simulink model "CrCtl_ShOff"  (R2016b)
settings: configuration reference "CodeGenConfigSet" (kept outside this file)
values from neighbouring files (symbols this model uses):
  CrCtl_aAccShOff_C = Calibration.Parameter    [init_CrCtl_ShOff.m]
  CrCtl_aDeclShOff_C = Calibration.Parameter    [init_CrCtl_ShOff.m]
  CrCtl_facDvtRelShOff_C = Calibration.Parameter    [init_CrCtl_ShOff.m]
  CrCtl_GearMin_C = Calibration.Parameter    [init_CrCtl_ShOff.m]
  CrCtl_nMaxShOff_C = Calibration.Parameter    [init_CrCtl_ShOff.m]
  CrCtl_nMinShOff_C = Calibration.Parameter    [init_CrCtl_ShOff.m]
  CRCTL_PAUSEENABLE_SY = uint8(0)    [init_CrCtl_ShOff.m]
  CrCtl_rTraV2NDvtAbsShOff_C = Calibration.Parameter    [init_CrCtl_ShOff.m]
  CrCtl_rTraV2NDvtShOff_C = Calibration.Parameter    [init_CrCtl_ShOff.m]
  CrCtl_rTraV2NSuspSync_C = Calibration.Parameter    [init_CrCtl_ShOff.m]
  CrCtl_stShOffCut_C = Calibration.Parameter    [init_CrCtl_ShOff.m]
  CrCtl_stShOffIrvrs_C = Calibration.Parameter    [init_CrCtl_ShOff.m]
  CrCtl_stShOffRvrs_C = Calibration.Parameter    [init_CrCtl_ShOff.m]
  CrCtl_stShOffRvrsDelVel_C = Calibration.Parameter    [init_CrCtl_ShOff.m]
  CrCtl_stShOffSlpCnstRmp_C = Calibration.Parameter    [init_CrCtl_ShOff.m]
  CrCtl_stShOffTimeCnstRmp_C = Calibration.Parameter    [init_CrCtl_ShOff.m]
  CrCtl_swtSuspEna_C = Calibration.Parameter    [init_CrCtl_ShOff.m]
  CrCtl_tiAccShOff_C = Calibration.Parameter    [init_CrCtl_ShOff.m]
  CrCtl_tiDeclShOff_C = Calibration.Parameter    [init_CrCtl_ShOff.m]
  CrCtl_tiDvtShOff_C = Calibration.Parameter    [init_CrCtl_ShOff.m]
  CrCtl_tiOverrideShOff_C = Calibration.Parameter    [init_CrCtl_ShOff.m]
  CrCtl_tiSuspClthPresMax_C = Calibration.Parameter    [init_CrCtl_ShOff.m]
  CrCtl_tiSuspMax_C = Calibration.Parameter    [init_CrCtl_ShOff.m]
  CrCtl_tiSuspSync_C = Calibration.Parameter    [init_CrCtl_ShOff.m]
  CrCtl_trqSpdGovInc_C = Calibration.Parameter    [init_CrCtl_ShOff.m]
  CrCtl_trqSpdGovMax_C = Calibration.Parameter    [init_CrCtl_ShOff.m]
  CrCtl_trqSpdGovRed_C = Calibration.Parameter    [init_CrCtl_ShOff.m]
  CrCtl_vDvtNegShOff_C = Calibration.Parameter    [init_CrCtl_ShOff.m]
  CrCtl_vDvtPosShOff_C = Calibration.Parameter    [init_CrCtl_ShOff.m]
  CrCtl_vDvtShOff_C = Calibration.Parameter    [init_CrCtl_ShOff.m]
  CrCtl_vMaxShOff_C = Calibration.Parameter    [init_CrCtl_ShOff.m]
  CrCtl_vMinShOff_C = Calibration.Parameter    [init_CrCtl_ShOff.m]
  TRQ_ENGINTV_SY = uint8(1)    [init_CrCtl_ShOff.m]
  VEL_ZERO = fi(0,VehSpeed_km_h)    [init_CrCtl_ShOff.m]
undefined symbols (not defined in the file or in its folder): CrCtl_ShOff_DT, CrCtl_stLck_conv, CrCtl_stOpFunc_conv, CrCtl_stShOff_conv, CrCtl_stSub_conv, CrCUI_BttnState_conv, CruiseCtl_State_conv, EngState_conv, Switch_conv
libraries: simulink x80, CXLib x24
(part 2 of 2)

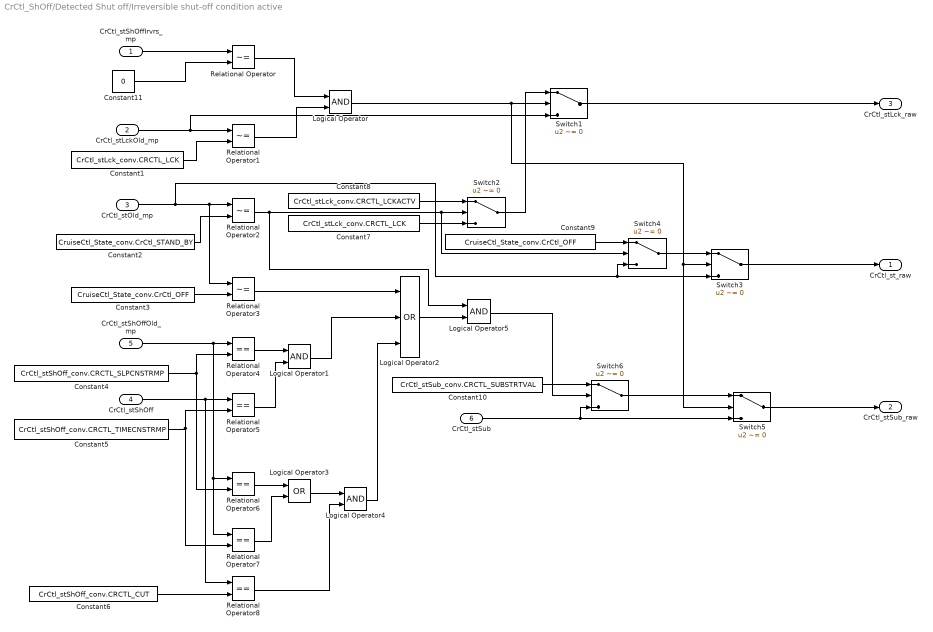
== system CrCtl_ShOff/Detected Shut off/Irreversible shut-off condition active ==
  CrCtl_stShOffIrvrs_mp : Inport
  CrCtl_stLckOld_mp : Inport  Port=2
  CrCtl_stOld_mp : Inport  Port=3
  CrCtl_stShOff : Inport  Port=4
  CrCtl_stShOffOld_mp : Inport  Port=5
  CrCtl_stSub : Inport  Port=6
  Constant1 : Constant  Value=CrCtl_stLck_conv.CRCTL_LCK
  Constant10 : Constant  Value=CrCtl_stSub_conv.CRCTL_SUBSTRTVAL
  Constant11 : Constant  Value=0  OutDataTypeStr=uint16
  Constant2 : Constant  Value=CruiseCtl_State_conv.CrCtl_STAND_BY
  Constant3 : Constant  Value=CruiseCtl_State_conv.CrCtl_OFF
  Constant4 : Constant  Value=CrCtl_stShOff_conv.CRCTL_SLPCNSTRMP
  Constant5 : Constant  Value=CrCtl_stShOff_conv.CRCTL_TIMECNSTRMP
  Constant6 : Constant  Value=CrCtl_stShOff_conv.CRCTL_CUT
  Constant7 : Constant  Value=CrCtl_stLck_conv.CRCTL_LCK
  Constant8 : Constant  Value=CrCtl_stLck_conv.CRCTL_LCKACTV
  Constant9 : Constant  Value=CruiseCtl_State_conv.CrCtl_OFF
  Logical Operator{,1,4..5} (4 alike) : Logic  AllPortsSameDT=off  OutDataTypeStr=boolean
  Logical Operator2 : Logic  Operator=OR  Inputs=3  AllPortsSameDT=off  OutDataTypeStr=boolean
  Logical Operator3 : Logic  Operator=OR  AllPortsSameDT=off  OutDataTypeStr=boolean
  Relational Operator{,1..3} (4 alike) : RelationalOperator  Operator=~=  OutDataTypeStr=boolean  RndMeth=Simplest
  Relational Operator{4..8} (5 alike) : RelationalOperator  Operator===  OutDataTypeStr=boolean  RndMeth=Simplest
  Switch{1..6} (6 alike) : Switch  Criteria=u2 ~= 0
  CrCtl_st_raw : Outport
  CrCtl_stSub_raw : Outport  Port=2
  CrCtl_stLck_raw : Outport  Port=3
  wires:
  CrCtl_stShOffIrvrs_mp/1 -> Relational Operator/1
  Constant11/1 -> Relational Operator/2
  Constant1/1 -> Relational Operator1/2
  Constant2/1 -> Relational Operator2/2
  Constant3/1 -> Relational Operator3/2
  CrCtl_stShOffOld_mp/1 -> Relational Operator7/1, Relational Operator6/1, Relational Operator4/1
  Constant4/1 -> Relational Operator6/2, Relational Operator4/2
  CrCtl_stShOff/1 -> Relational Operator8/1, Relational Operator5/1
  Constant5/1 -> Relational Operator7/2, Relational Operator5/2
  Constant6/1 -> Relational Operator8/2
  Relational Operator/1 -> Logical Operator/1
  Relational Operator1/1 -> Logical Operator/2
  Switch1/1 -> CrCtl_stLck_raw/1
  CrCtl_stLckOld_mp/1 -> Switch1/3, Relational Operator1/1
  Relational Operator2/1 -> Switch4/2, Switch2/2, Logical Operator5/1
  Switch2/1 -> Switch1/1
  Constant7/1 -> Switch2/3
  Constant8/1 -> Switch2/1
  Relational Operator4/1 -> Logical Operator1/1
  Relational Operator5/1 -> Logical Operator1/2
  Logical Operator1/1 -> Logical Operator2/2
  Relational Operator3/1 -> Logical Operator2/1
  Relational Operator6/1 -> Logical Operator3/1
  Relational Operator7/1 -> Logical Operator3/2
  Relational Operator8/1 -> Logical Operator4/2
  Logical Operator3/1 -> Logical Operator4/1
  Logical Operator4/1 -> Logical Operator2/3
  Logical Operator2/1 -> Logical Operator5/2
  Switch3/1 -> CrCtl_st_raw/1
  CrCtl_stOld_mp/1 -> Switch4/3, Switch3/3, Relational Operator3/1, Relational Operator2/1
  Switch4/1 -> Switch3/1
  Logical Operator/1 -> Switch5/2, Switch3/2, Switch1/2
  Switch5/1 -> CrCtl_stSub_raw/1
  CrCtl_stSub/1 -> Switch5/3, Switch6/3
  Switch6/1 -> Switch5/1
  Constant9/1 -> Switch4/1
  Logical Operator5/1 -> Switch6/2
  Constant10/1 -> Switch6/1

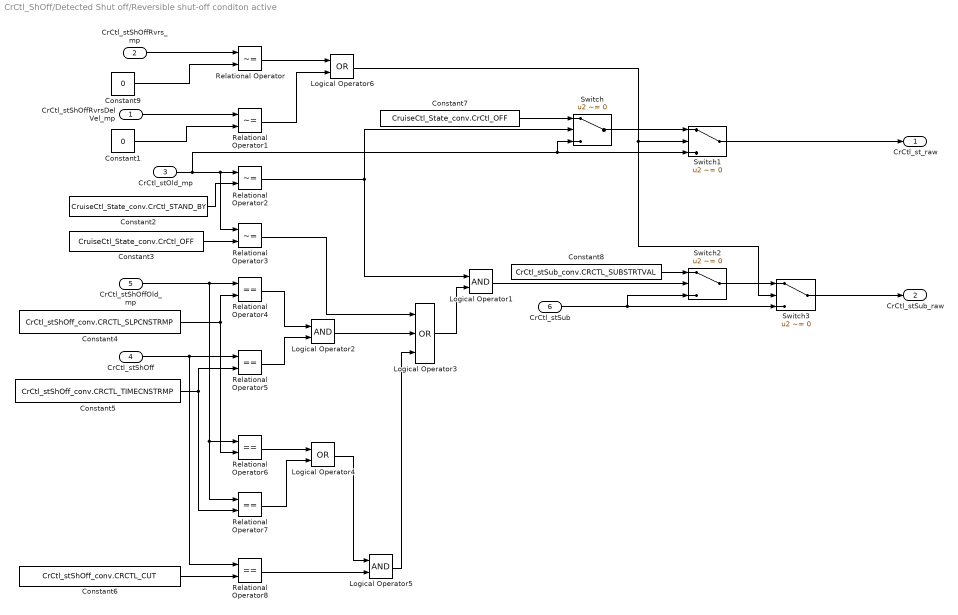
== system CrCtl_ShOff/Detected Shut off/Reversible shut-off conditon active ==
  CrCtl_stShOffRvrsDelVel_mp : Inport
  CrCtl_stShOffRvrs_mp : Inport  Port=2
  CrCtl_stOld_mp : Inport  Port=3
  CrCtl_stShOff : Inport  Port=4
  CrCtl_stShOffOld_mp : Inport  Port=5
  CrCtl_stSub : Inport  Port=6
  Constant1 : Constant  Value=0  OutDataTypeStr=uint16
  Constant2 : Constant  Value=CruiseCtl_State_conv.CrCtl_STAND_BY
  Constant3 : Constant  Value=CruiseCtl_State_conv.CrCtl_OFF
  Constant4 : Constant  Value=CrCtl_stShOff_conv.CRCTL_SLPCNSTRMP
  Constant5 : Constant  Value=CrCtl_stShOff_conv.CRCTL_TIMECNSTRMP
  Constant6 : Constant  Value=CrCtl_stShOff_conv.CRCTL_CUT
  Constant7 : Constant  Value=CruiseCtl_State_conv.CrCtl_OFF
  Constant8 : Constant  Value=CrCtl_stSub_conv.CRCTL_SUBSTRTVAL
  Constant9 : Constant  Value=0  OutDataTypeStr=uint16
  Logical Operator1 : Logic  AllPortsSameDT=off  OutDataTypeStr=boolean
  Logical Operator2 : Logic  AllPortsSameDT=off  OutDataTypeStr=boolean
  Logical Operator3 : Logic  Operator=OR  Inputs=3  AllPortsSameDT=off  OutDataTypeStr=boolean
  Logical Operator4 : Logic  Operator=OR  AllPortsSameDT=off  OutDataTypeStr=boolean
  Logical Operator5 : Logic  AllPortsSameDT=off  OutDataTypeStr=boolean
  Logical Operator6 : Logic  Operator=OR  AllPortsSameDT=off  OutDataTypeStr=boolean
  Relational Operator{,1..3} (4 alike) : RelationalOperator  Operator=~=  OutDataTypeStr=boolean  RndMeth=Simplest
  Relational Operator{4..8} (5 alike) : RelationalOperator  Operator===  OutDataTypeStr=boolean  RndMeth=Simplest
  Switch{,1..3} (4 alike) : Switch  Criteria=u2 ~= 0
  CrCtl_st_raw : Outport
  CrCtl_stSub_raw : Outport  Port=2
  wires:
  CrCtl_stShOffRvrs_mp/1 -> Relational Operator/1
  Constant9/1 -> Relational Operator/2
  CrCtl_stShOffRvrsDelVel_mp/1 -> Relational Operator1/1
  Constant1/1 -> Relational Operator1/2
  Constant2/1 -> Relational Operator2/2
  Constant3/1 -> Relational Operator3/2
  CrCtl_stShOffOld_mp/1 -> Relational Operator7/1, Relational Operator6/1, Relational Operator4/1
  Constant4/1 -> Relational Operator4/2, Relational Operator6/2
  CrCtl_stShOff/1 -> Relational Operator8/1, Relational Operator5/1
  Constant5/1 -> Relational Operator5/2, Relational Operator7/2
  Constant6/1 -> Relational Operator8/2
  Relational Operator/1 -> Logical Operator6/1
  Relational Operator1/1 -> Logical Operator6/2
  Relational Operator2/1 -> Logical Operator1/1, Switch/2
  Switch/1 -> Switch1/1
  Switch1/1 -> CrCtl_st_raw/1
  CrCtl_stOld_mp/1 -> Switch/3, Switch1/3, Relational Operator3/1, Relational Operator2/1
  Constant7/1 -> Switch/1
  Relational Operator4/1 -> Logical Operator2/1
  Relational Operator5/1 -> Logical Operator2/2
  Logical Operator2/1 -> Logical Operator3/2
  Relational Operator3/1 -> Logical Operator3/1
  Relational Operator6/1 -> Logical Operator4/1
  Relational Operator7/1 -> Logical Operator4/2
  Relational Operator8/1 -> Logical Operator5/2
  Logical Operator4/1 -> Logical Operator5/1
  Logical Operator5/1 -> Logical Operator3/3
  Logical Operator3/1 -> Logical Operator1/2
  Logical Operator1/1 -> Switch2/2
  Switch2/1 -> Switch3/1
  Switch3/1 -> CrCtl_stSub_raw/1
  CrCtl_stSub/1 -> Switch3/3, Switch2/3
  Constant8/1 -> Switch2/1
  Logical Operator6/1 -> Switch3/2, Switch1/2

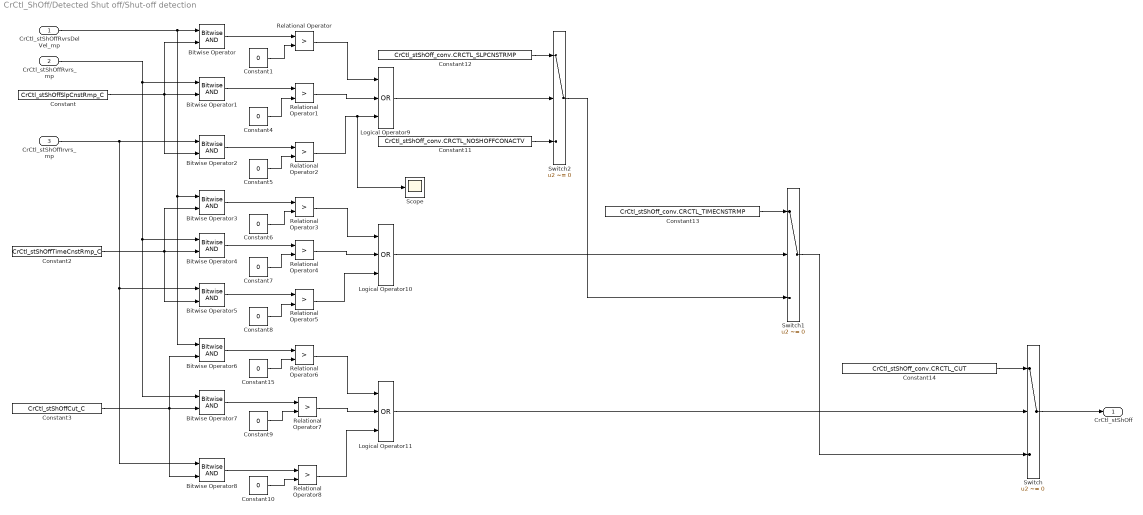
== system CrCtl_ShOff/Detected Shut off/Shut-off detection ==
  CrCtl_stShOffRvrsDelVel_mp : Inport
  CrCtl_stShOffRvrs_mp : Inport  Port=2
  CrCtl_stShOffIrvrs_mp : Inport  Port=3
  Bitwise Operator{,1..8} (9 alike) : simulink/Logic and Bit Operations/Bitwise Operator  logicop=AND  UseBitMask=off  NumInputPorts=2  BitMask=bin2dec('11011001')  BitMaskRealWorld=Stored Integer
  Constant : Constant  Value=CrCtl_stShOffSlpCnstRmp_C
  Constant{1,4..10,15} (9 alike) : Constant  Value=0  OutDataTypeStr=uint32
  Constant11 : Constant  Value=CrCtl_stShOff_conv.CRCTL_NOSHOFFCONACTV
  Constant12 : Constant  Value=CrCtl_stShOff_conv.CRCTL_SLPCNSTRMP
  Constant13 : Constant  Value=CrCtl_stShOff_conv.CRCTL_TIMECNSTRMP
  Constant14 : Constant  Value=CrCtl_stShOff_conv.CRCTL_CUT
  Constant2 : Constant  Value=CrCtl_stShOffTimeCnstRmp_C
  Constant3 : Constant  Value=CrCtl_stShOffCut_C
  Logical Operator10 : Logic  Operator=OR  Inputs=3  AllPortsSameDT=off  OutDataTypeStr=boolean
  Logical Operator11 : Logic  Operator=OR  Inputs=3  AllPortsSameDT=off  OutDataTypeStr=boolean
  Logical Operator9 : Logic  Operator=OR  Inputs=3  AllPortsSameDT=off  OutDataTypeStr=boolean
  Relational Operator{,1..8} (9 alike) : RelationalOperator  Operator=>  OutDataTypeStr=boolean  RndMeth=Simplest
  Scope : Scope
  Switch : Switch  Criteria=u2 ~= 0
  Switch1 : Switch  Criteria=u2 ~= 0
  Switch2 : Switch  Criteria=u2 ~= 0
  CrCtl_stShOff : Outport
  wires:
  Constant3/1 -> Bitwise Operator8/2, Bitwise Operator7/2, Bitwise Operator6/2
  CrCtl_stShOffRvrsDelVel_mp/1 -> Bitwise Operator6/1, Bitwise Operator3/1, Bitwise Operator/1
  CrCtl_stShOffRvrs_mp/1 -> Bitwise Operator7/1, Bitwise Operator4/1, Bitwise Operator1/1
  CrCtl_stShOffIrvrs_mp/1 -> Bitwise Operator8/1, Bitwise Operator5/1, Bitwise Operator2/1
  Constant/1 -> Bitwise Operator2/2, Bitwise Operator1/2, Bitwise Operator/2
  Constant2/1 -> Bitwise Operator5/2, Bitwise Operator4/2, Bitwise Operator3/2
  Constant1/1 -> Relational Operator/2
  Bitwise Operator/1 -> Relational Operator/1
  Bitwise Operator1/1 -> Relational Operator1/1
  Constant4/1 -> Relational Operator1/2
  Bitwise Operator2/1 -> Relational Operator2/1
  Constant5/1 -> Relational Operator2/2
  Bitwise Operator3/1 -> Relational Operator3/1
  Constant6/1 -> Relational Operator3/2
  Bitwise Operator4/1 -> Relational Operator4/1
  Constant7/1 -> Relational Operator4/2
  Bitwise Operator5/1 -> Relational Operator5/1
  Constant8/1 -> Relational Operator5/2
  Bitwise Operator6/1 -> Relational Operator6/1
  Constant15/1 -> Relational Operator6/2
  Bitwise Operator7/1 -> Relational Operator7/1
  Constant9/1 -> Relational Operator7/2
  Bitwise Operator8/1 -> Relational Operator8/1
  Constant10/1 -> Relational Operator8/2
  Relational Operator1/1 -> Logical Operator9/2
  Relational Operator/1 -> Logical Operator9/1
  Relational Operator2/1 -> Scope/1, Logical Operator9/3
  Relational Operator4/1 -> Logical Operator10/2
  Relational Operator3/1 -> Logical Operator10/1
  Relational Operator5/1 -> Logical Operator10/3
  Relational Operator7/1 -> Logical Operator11/2
  Relational Operator6/1 -> Logical Operator11/1
  Relational Operator8/1 -> Logical Operator11/3
  Constant13/1 -> Switch1/1
  Switch/1 -> CrCtl_stShOff/1
  Constant14/1 -> Switch/1
  Constant12/1 -> Switch2/1
  Logical Operator9/1 -> Switch2/2
  Logical Operator10/1 -> Switch1/2
  Logical Operator11/1 -> Switch/2
  Switch1/1 -> Switch/3
  Switch2/1 -> Switch1/3
  Constant11/1 -> Switch2/3

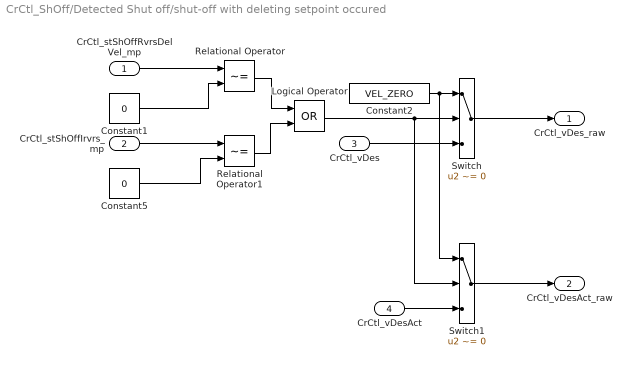
== system CrCtl_ShOff/Detected Shut off/shut-off with deleting setpoint occured ==
  CrCtl_stShOffRvrsDelVel_mp : Inport
  CrCtl_stShOffIrvrs_mp : Inport  Port=2
  CrCtl_vDes : Inport  Port=3
  CrCtl_vDesAct : Inport  Port=4
  Constant1 : Constant  Value=0  OutDataTypeStr=uint16
  Constant2 : Constant  Value=VEL_ZERO
  Constant5 : Constant  Value=0  OutDataTypeStr=uint16
  Logical Operator : Logic  Operator=OR  AllPortsSameDT=off  OutDataTypeStr=boolean
  Relational Operator : RelationalOperator  Operator=~=  OutDataTypeStr=boolean  RndMeth=Simplest
  Relational Operator1 : RelationalOperator  Operator=~=  OutDataTypeStr=boolean  RndMeth=Simplest
  Switch : Switch  Criteria=u2 ~= 0
  Switch1 : Switch  Criteria=u2 ~= 0
  CrCtl_vDes_raw : Outport
  CrCtl_vDesAct_raw : Outport  Port=2
  wires:
  CrCtl_stShOffRvrsDelVel_mp/1 -> Relational Operator/1
  Constant1/1 -> Relational Operator/2
  CrCtl_stShOffIrvrs_mp/1 -> Relational Operator1/1
  Constant5/1 -> Relational Operator1/2
  Relational Operator/1 -> Logical Operator/1
  Relational Operator1/1 -> Logical Operator/2
  Switch/1 -> CrCtl_vDes_raw/1
  Constant2/1 -> Switch1/1, Switch/1
  Logical Operator/1 -> Switch1/2, Switch/2
  CrCtl_vDes/1 -> Switch/3
  CrCtl_vDesAct/1 -> Switch1/3
  Switch1/1 -> CrCtl_vDesAct_raw/1

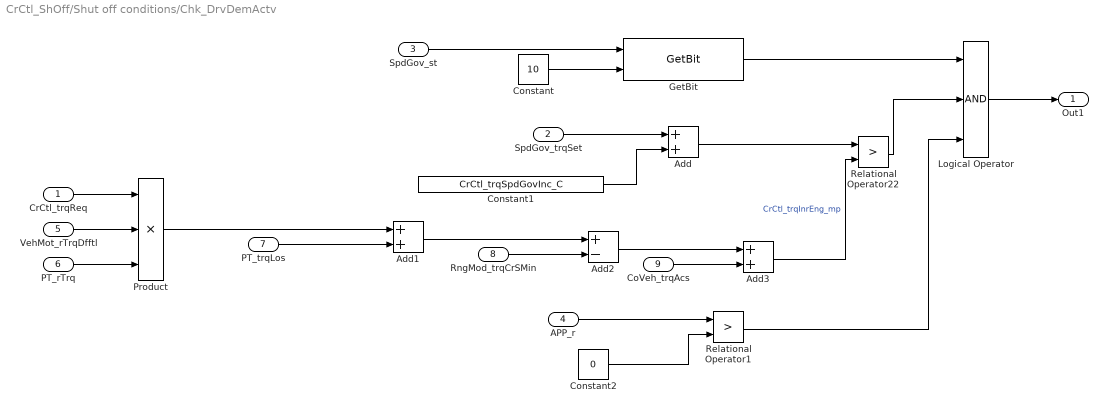
== system CrCtl_ShOff/Shut off conditions/Chk_DrvDemActv ==
  CrCtl_trqReq : Inport
  SpdGov_trqSet : Inport  Port=2
  SpdGov_st : Inport  Port=3
  APP_r : Inport  Port=4
  VehMot_rTrqDfftl : Inport  Port=5
  PT_rTrq : Inport  Port=6
  PT_trqLos : Inport  Port=7
  RngMod_trqCrSMin : Inport  Port=8
  CoVeh_trqAcs : Inport  Port=9
  Add : Sum
  Add1 : Sum
  Add2 : Sum  Inputs=+-
  Add3 : Sum
  Constant : Constant  Value=10  OutDataTypeStr=uint8
  Constant1 : Constant  Value=CrCtl_trqSpdGovInc_C
  Constant2 : Constant  Value=0
  GetBit : CXLib/GetBit  dataTypeString=uint16  dataLength=0
      settings: AttributesFormatString=Get bit from %<dataTypeString>
  Logical Operator : Logic  Inputs=3  AllPortsSameDT=off  OutDataTypeStr=boolean
  Product : Product  Inputs=3  OutDataTypeStr=Trq_Nm
  Relational Operator1 : RelationalOperator  Operator=>  OutDataTypeStr=boolean  RndMeth=Simplest
  Relational Operator22 : RelationalOperator  Operator=>  OutDataTypeStr=boolean  RndMeth=Simplest
  Out1 : Outport
  wires:
  Constant/1 -> GetBit/2
  SpdGov_st/1 -> GetBit/1
  GetBit/1 -> Logical Operator/1
  Constant1/1 -> Add/2
  SpdGov_trqSet/1 -> Add/1
  Add/1 -> Relational Operator22/1
  Relational Operator22/1 -> Logical Operator/2
  CrCtl_trqReq/1 -> Product/1
  VehMot_rTrqDfftl/1 -> Product/2
  PT_rTrq/1 -> Product/3
  Add2/1 -> Add3/1
  Product/1 -> Add1/1
  PT_trqLos/1 -> Add1/2
  Add1/1 -> Add2/1
  RngMod_trqCrSMin/1 -> Add2/2
  CoVeh_trqAcs/1 -> Add3/2
  Add3/1 -> Relational Operator22/2  "CrCtl_trqInrEng_mp"
  APP_r/1 -> Relational Operator1/1
  Constant2/1 -> Relational Operator1/2
  Relational Operator1/1 -> Logical Operator/3
  Logical Operator/1 -> Out1/1

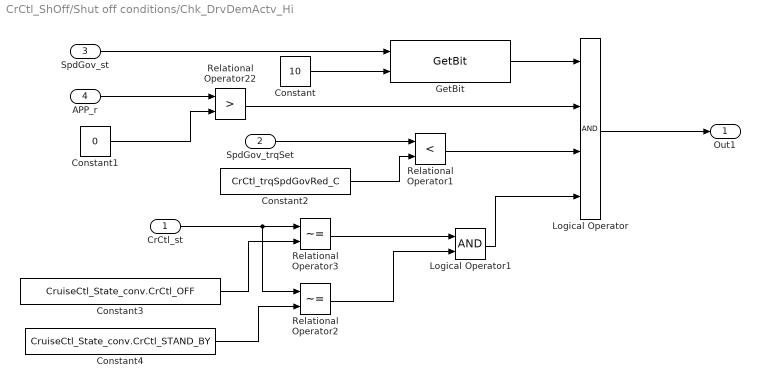
== system CrCtl_ShOff/Shut off conditions/Chk_DrvDemActv_Hi ==
  CrCtl_st : Inport
  SpdGov_trqSet : Inport  Port=2
  SpdGov_st : Inport  Port=3
  APP_r : Inport  Port=4
  Constant : Constant  Value=10  OutDataTypeStr=uint8
  Constant1 : Constant  Value=0
  Constant2 : Constant  Value=CrCtl_trqSpdGovRed_C
  Constant3 : Constant  Value=CruiseCtl_State_conv.CrCtl_OFF
  Constant4 : Constant  Value=CruiseCtl_State_conv.CrCtl_STAND_BY
  GetBit : CXLib/GetBit  dataTypeString=uint16  dataLength=0
      settings: AttributesFormatString=Get bit from %<dataTypeString>
  Logical Operator : Logic  Inputs=4'  AllPortsSameDT=off  OutDataTypeStr=boolean
  Logical Operator1 : Logic  AllPortsSameDT=off  OutDataTypeStr=boolean
  Relational Operator1 : RelationalOperator  Operator=<  OutDataTypeStr=boolean  RndMeth=Simplest
  Relational Operator2 : RelationalOperator  Operator=~=  OutDataTypeStr=boolean  RndMeth=Simplest
  Relational Operator22 : RelationalOperator  Operator=>  OutDataTypeStr=boolean  RndMeth=Simplest
  Relational Operator3 : RelationalOperator  Operator=~=  OutDataTypeStr=boolean  RndMeth=Simplest
  Out1 : Outport
  wires:
  Constant/1 -> GetBit/2
  SpdGov_st/1 -> GetBit/1
  GetBit/1 -> Logical Operator/1
  APP_r/1 -> Relational Operator22/1
  Constant1/1 -> Relational Operator22/2
  Relational Operator22/1 -> Logical Operator/2
  Logical Operator/1 -> Out1/1
  SpdGov_trqSet/1 -> Relational Operator1/1
  Constant2/1 -> Relational Operator1/2
  Relational Operator1/1 -> Logical Operator/3
  CrCtl_st/1 -> Relational Operator2/1, Relational Operator3/1
  Constant3/1 -> Relational Operator3/2
  Constant4/1 -> Relational Operator2/2
  Relational Operator3/1 -> Logical Operator1/1
  Relational Operator2/1 -> Logical Operator1/2
  Logical Operator1/1 -> Logical Operator/4

== system CrCtl_ShOff/Shut off conditions/EBC1//VDC1 Shut off conditons ==
  Anti-Lock braking Engine Control : Subsystem
  Drag Torque Control Active : Subsystem
  Logical Operator : Logic  Operator=OR  Inputs=8  AllPortsSameDT=off  OutDataTypeStr=boolean
  Roll Over Prv Brake : Subsystem
  Roll Over Prv Engine : Subsystem
  TCS Brake Control : Subsystem
  TCS Engine Control : Subsystem
  Yaw Control Brake : Subsystem
  Yaw Control Engine : Subsystem
  Out1 : Outport
  wires:
  TCS Brake Control/1(Out1) -> Logical Operator/1
  TCS Engine Control/1(Out2) -> Logical Operator/2
  Drag Torque Control Active/1(Out1) -> Logical Operator/3
  Yaw Control Brake/1(Out1) -> Logical Operator/4
  Yaw Control Engine/1(Out1) -> Logical Operator/5
  Roll Over Prv Brake/1(Out1) -> Logical Operator/6
  Roll Over Prv Engine/1(Out1) -> Logical Operator/7
  Anti-Lock braking Engine Control/1(Out1) -> Logical Operator/8
  Logical Operator/1 -> Out1/1

== system CrCtl_ShOff/Suspend function/Suspend function active ==
  In1 : Inport
  In2 : Inport  Port=2
  Enable : EnablePort
  Clutch is pressed : Subsystem
  "Clutch is released " : Subsystem
  Logical Operator1 : Logic  Operator=NOT  AllPortsSameDT=off  OutDataTypeStr=boolean
  Merge : Merge
  CrCtl_rTraV2NSusp : Outport
  CrCtl_rTraV2NBeg : Outport  Port=2
  CrCtl_stSuspAct : Outport  Port=3
  wires:
  In1/1 -> Logical Operator1/1, Clutch is pressed/Enable
  In2/1 -> "Clutch is released "/1(PT_rTraV2N), Clutch is pressed/1(PT_rTraV2N)
  Clutch is pressed/1(CrCtl_stSuspAct) -> Merge/2
  "Clutch is released "/2(CrCtl_stSuspAct) -> Merge/1
  "Clutch is released "/1(CrCtl_rTraV2NBeg) -> CrCtl_rTraV2NBeg/1
  Clutch is pressed/2(CrCtl_rTraV2NSusp) -> "Clutch is released "/2(rTraV2NSusp)
  Merge/1 -> CrCtl_stSuspAct/1
  Logical Operator1/1 -> "Clutch is released "/Enable
  "Clutch is released "/3(CrCtl_rTraV2NSusp) -> CrCtl_rTraV2NSusp/1

== system CrCtl_ShOff/Shut off conditions/EBC1//VDC1 Shut off conditons/Anti-Lock braking Engine Control ==
  Constant : Constant  Value=0
  Out1 : Outport
  wires:
  Constant/1 -> Out1/1

== system CrCtl_ShOff/Shut off conditions/EBC1//VDC1 Shut off conditons/Drag Torque Control Active ==
  Constant : Constant  Value=0
  Out1 : Outport
  wires:
  Constant/1 -> Out1/1

== system CrCtl_ShOff/Shut off conditions/EBC1//VDC1 Shut off conditons/Roll Over Prv Brake ==
  Constant : Constant  Value=0
  Out1 : Outport
  wires:
  Constant/1 -> Out1/1

== system CrCtl_ShOff/Shut off conditions/EBC1//VDC1 Shut off conditons/Roll Over Prv Engine ==
  Constant : Constant  Value=0
  Out1 : Outport
  wires:
  Constant/1 -> Out1/1

== system CrCtl_ShOff/Shut off conditions/EBC1//VDC1 Shut off conditons/TCS Brake Control ==
  Constant : Constant  Value=0
  Out1 : Outport
  wires:
  Constant/1 -> Out1/1

== system CrCtl_ShOff/Shut off conditions/EBC1//VDC1 Shut off conditons/TCS Engine Control ==
  Constant : Constant  Value=0
  Out2 : Outport
  wires:
  Constant/1 -> Out2/1

== system CrCtl_ShOff/Shut off conditions/EBC1//VDC1 Shut off conditons/Yaw Control Brake ==
  Constant : Constant  Value=0
  Out1 : Outport
  wires:
  Constant/1 -> Out1/1

== system CrCtl_ShOff/Shut off conditions/EBC1//VDC1 Shut off conditons/Yaw Control Engine ==
  Constant : Constant  Value=0
  Out1 : Outport
  wires:
  Constant/1 -> Out1/1

== system CrCtl_ShOff/Suspend function/Suspend function active/Clutch is pressed ==
  PT_rTraV2N : Inport
  Enable : EnablePort  ShowOutputPort=on
  Constant2 : Constant  Value=CrCtl_ShOff_DT
  Constant3 : Constant  Value=CrCtl_tiSuspClthPresMax_C
  EdgeFalling : CXLib/EdgeFalling
  Relational Operator : RelationalOperator  Operator=<=  OutDataTypeStr=boolean  RndMeth=Simplest
  Timer_Up : CXLib/Timer_Up
  CrCtl_stSuspAct : Outport
  CrCtl_rTraV2NSusp : Outport  Port=2
  wires:
  Enable/1 -> EdgeFalling/1, Timer_Up/1
  Constant2/1 -> Timer_Up/3
  EdgeFalling/1 -> Timer_Up/2
  Timer_Up/1 -> Relational Operator/1
  Constant3/1 -> Relational Operator/2
  Relational Operator/1 -> CrCtl_stSuspAct/1
  PT_rTraV2N/1 -> CrCtl_rTraV2NSusp/1

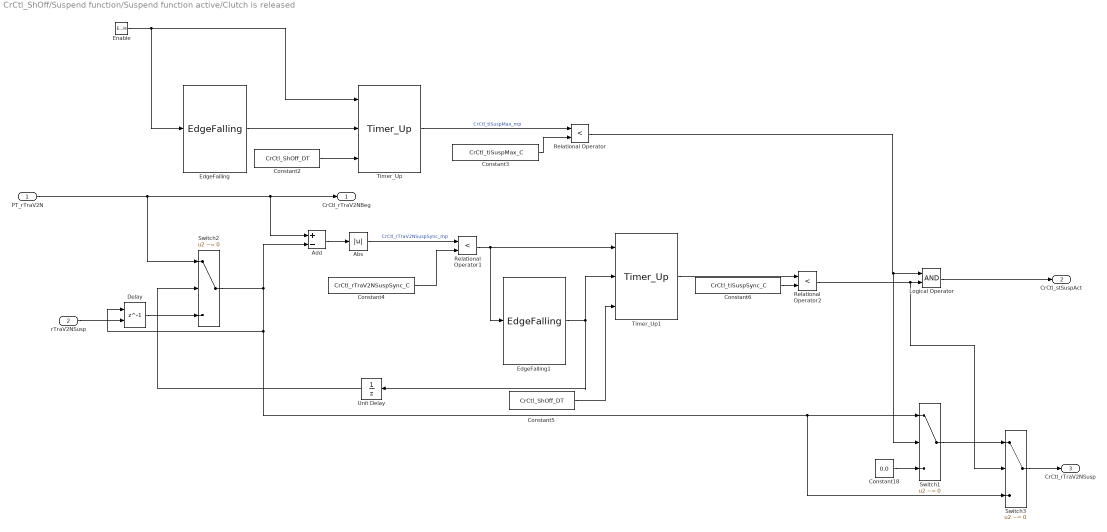
== system CrCtl_ShOff/Suspend function/Suspend function active/Clutch is released  ==
  PT_rTraV2N : Inport
  rTraV2NSusp : Inport  Port=2
  Enable : EnablePort  ShowOutputPort=on
  Abs : Abs
  Add : Sum  Inputs=+-
  Constant18 : Constant  Value=0.0  OutDataTypeStr=Tra_V2N_km_h_rpm
  Constant2 : Constant  Value=CrCtl_ShOff_DT
  Constant3 : Constant  Value=CrCtl_tiSuspMax_C
  Constant4 : Constant  Value=CrCtl_rTraV2NSuspSync_C
  Constant5 : Constant  Value=CrCtl_ShOff_DT
  Constant6 : Constant  Value=CrCtl_tiSuspSync_C
  Delay : Delay  DelayLength=1  InitialConditionSource=Input port
      settings: InputPortMap=u0,p4
  EdgeFalling : CXLib/EdgeFalling
  EdgeFalling1 : CXLib/EdgeFalling
  Logical Operator : Logic  AllPortsSameDT=off  OutDataTypeStr=boolean
  Relational Operator : RelationalOperator  Operator=<  OutDataTypeStr=boolean  RndMeth=Simplest
  Relational Operator1 : RelationalOperator  Operator=<  OutDataTypeStr=boolean  RndMeth=Simplest
  Relational Operator2 : RelationalOperator  Operator=<  OutDataTypeStr=boolean  RndMeth=Simplest
  Switch1 : Switch  Criteria=u2 ~= 0
  Switch2 : Switch  Criteria=u2 ~= 0
  Switch3 : Switch  Criteria=u2 ~= 0
  Timer_Up : CXLib/Timer_Up
  Timer_Up1 : CXLib/Timer_Up
  Unit Delay : UnitDelay  SampleTime=-1
  CrCtl_rTraV2NBeg : Outport
  CrCtl_stSuspAct : Outport  Port=2
  CrCtl_rTraV2NSusp : Outport  Port=3
  wires:
  Enable/1 -> EdgeFalling/1, Timer_Up/1
  Constant2/1 -> Timer_Up/3
  EdgeFalling/1 -> Timer_Up/2
  Timer_Up/1 -> Relational Operator/1  "CrCtl_tiSuspMax_mp"
  Constant3/1 -> Relational Operator/2
  PT_rTraV2N/1 -> Switch2/1, Add/1, CrCtl_rTraV2NBeg/1
  Add/1 -> Abs/1
  Abs/1 -> Relational Operator1/1  "CrCtl_rTraV2NSuspSync_mp"
  Constant4/1 -> Relational Operator1/2
  Relational Operator2/1 -> Switch3/2, Logical Operator/2
  Constant5/1 -> Timer_Up1/3
  Timer_Up1/1 -> Relational Operator2/1
  Constant6/1 -> Relational Operator2/2
  Relational Operator/1 -> Switch1/2, Logical Operator/1
  Relational Operator1/1 -> Timer_Up1/1, EdgeFalling1/1
  Logical Operator/1 -> CrCtl_stSuspAct/1
  EdgeFalling1/1 -> Timer_Up1/2, Unit Delay/1
  rTraV2NSusp/1 -> Delay/2
  Switch2/1 -> Switch3/3, Switch1/1, Delay/1, Add/2
  Delay/1 -> Switch2/3
  Constant18/1 -> Switch1/3
  Switch1/1 -> Switch3/1
  Switch3/1 -> CrCtl_rTraV2NSusp/1
  Unit Delay/1 -> Switch2/2
